simulink library "NeuroMuscularLibrary"  (R2019b)
settings: Solver=ode45  StartTime=0.0  StopTime=10.0  RelTol=1e-3  EnableMultiTasking=on
values from neighbouring files (symbols this model uses):
  a_18_19 = 116    [Prosthesis3R60Params.m]
  a_18_21 = 34    [Prosthesis3R60Params.m]
  a_2_3 = 18    [Prosthesis3R60Params.m]
  angle_offset = 0    [Prosthesis3R60Params.m]
  ankle_height = 0.08    [BodyMechParams.m]
  c = 0.05    [BodyMechParams.m]
  c_jointstop = 0.3 / (pi/180)    (= 17.1887338539)    [BodyMechParams.m]
  c_stance_comp_a0 = 885.0653    [Prosthesis3R60Params.m]
  c_stance_comp_a1 = 2.1443    [Prosthesis3R60Params.m]
  cg14 = 1/2*L14    (= 0.0475)    [Prosthesis3R60Params.m]
  cg25 = (5.45/11.05)*L25    (= 0.0379527149321)    [Prosthesis3R60Params.m]
  cg3 = (3.6/10.4)*L3    (= 0.0306346153846)    [Prosthesis3R60Params.m]
  d_fBall = 0.1    [BodyMechParams.m]
  d_fHeel = 0.05    [BodyMechParams.m]
  deltaLegAngleThr = 8*pi/180    (= 0.13962634016)    [CMGParams.m]
  DeltaThRef = 2e-3    (= 0.002)    [BodyMechParams.m]
  dt_visual = 0.001    [Prosthesis3R60Params.m]
  eref = 0.04    [BodyMechParams.m]
  Fmax = 4000    [MuscleEnergyTest.m]
  FmaxGLU = 1500    [BodyMechParams.m]
  footBallToAnkleDist = 0.16    [BodyMechParams.m]
  footBallToCenterDist = footLength/2    (= 0.1)    [BodyMechParams.m]
  footBallToHeelDist = footLength    (= 0.2)    [BodyMechParams.m]
  footCenterToCGDist = 0.14 - footBallToCenterDist    (= 0.04)    [BodyMechParams.m]
  footInertia = 0.005    [BodyMechParams.m]
  footLength = 0.2    [BodyMechParams.m]
  footMass = 1.25    [BodyMechParams.m]
  FT = 20    [MuscleEnergyTest.m]
  FT_GLU = 47.6    [BodyMechParams.m]
  g = 9.80665    [BodyMechParams.m]
  groundTheta = [atan(diff(groundZ)./diff(groundX)), 0]    [generateGround.m]
  groundZ = groundZ * stepSize/(largestStep+eps)    [generateGround.m]
  hatCenterToCGDist = 0.35 - hatHipToCenterDistLen    (= -0.05)    [BodyMechParams.m]
  hatHipToCenterDistLen = hatLength/2    (= 0.4)    [BodyMechParams.m]
  hatInertia = 3    [BodyMechParams.m]
  hatLeftHipToCenterDistWidth = .15    (= 0.15)    [BodyMechParams.m]
  hatLength = 0.8    [BodyMechParams.m]
  hatMass = 53.5    [BodyMechParams.m]
  hatThickness = 0.2    [BodyMechParams.m]
  hatWidth = 0.4    [BodyMechParams.m]
  J1011 = (4130)*1e-9    (= 4.13e-06)    [Prosthesis3R60Params.m]
  J1415 = (1.18*1e5)*1e-9    (= 0.000118)    [Prosthesis3R60Params.m]
  J18192021 = (6.86*1e4)*1e-9    (= 6.86e-05)    [Prosthesis3R60Params.m]
  J2526 = (3.59*1e4)*1e-9    (= 3.59e-05)    [Prosthesis3R60Params.m]
  J3467 = (25.96*1e4)*1e-9    (= 0.0002596)    [Prosthesis3R60Params.m]
  K = 5    [BodyMechParams.m]
  k_gn = k_gn/2    (= 39226.6)    [BodyMechParams.m]
  k_gt = k_gt/2    (= 39226.6)    [BodyMechParams.m]
  k_pressure = hatMass * g / DeltaThRef    (= 262327.8875)    [BodyMechParams.m]
  k_stance = 130000    [Prosthesis3R60Params.m]
  k_swing = 18750    [Prosthesis3R60Params.m]
  L0_stance = 0.08925    [Prosthesis3R60Params.m]
  L0_swing = 0.0896    [Prosthesis3R60Params.m]
  L10 = 7.9*1e-3    (= 0.0079)    [Prosthesis3R60Params.m]
  L11 = 3.3*1e-3    (= 0.0033)    [Prosthesis3R60Params.m]
  L14 = 95*1e-3    (= 0.095)    [Prosthesis3R60Params.m]
  L15 = 8.2*1e-3    (= 0.0082)    [Prosthesis3R60Params.m]
  L18 = 25.1*1e-3    (= 0.0251)    [Prosthesis3R60Params.m]
  L19 = 17.7*1e-3    (= 0.0177)    [Prosthesis3R60Params.m]
  L20 = 26*1e-3    (= 0.026)    [Prosthesis3R60Params.m]
  L21 = 1.7*1e-3    (= 0.0017)    [Prosthesis3R60Params.m]
  L25 = 76.95*1e-3    (= 0.07695)    [Prosthesis3R60Params.m]
  L26 = 2.8*1e-3    (= 0.0028)    [Prosthesis3R60Params.m]
  L3 = 88.5*1e-3    (= 0.0885)    [Prosthesis3R60Params.m]
  L4 = 1.7*1e-3    (= 0.0017)    [Prosthesis3R60Params.m]
  L6 = 40.25*1e-3    (= 0.04025)    [Prosthesis3R60Params.m]
  L7 = 14.9*1e-3    (= 0.0149)    [Prosthesis3R60Params.m]
  leg_l = [(thighLength - ankle_height/2) (shankLength - ankle_height/2)]    [BodyMechParams.m]
  legAngleSpeedMax = 10    [CMGParams.m]
  lopt = 0.055    [MuscleEnergyTest.m]
  loptBFSH = 0.12    [BodyMechParams.m]
  loptGAS = 0.05    [BodyMechParams.m]
  loptGLU = 0.11    [BodyMechParams.m]
  loptHAB = 0.09    [BodyMechParams.m]
  loptHAD = 0.10    (= 0.1)    [BodyMechParams.m]
  loptHAM = 0.10    (= 0.1)    [BodyMechParams.m]
  loptHFL = 0.11    [BodyMechParams.m]
  loptRF = 0.08    [BodyMechParams.m]
  loptSOL = 0.04    [BodyMechParams.m]
  loptTA = 0.06    [BodyMechParams.m]
  loptVAS = 0.08    [BodyMechParams.m]
  lslack = 0.245    [MuscleEnergyTest.m]
  lslackBFSH = 0.10    (= 0.1)    [BodyMechParams.m]
  lslackGAS = 0.40    (= 0.4)    [BodyMechParams.m]
  lslackGLU = 0.13    [BodyMechParams.m]
  lslackHAB = 0.07    [BodyMechParams.m]
  lslackHAD = 0.18    [BodyMechParams.m]
  lslackHAM = 0.31    [BodyMechParams.m]
  lslackHFL = 0.10    (= 0.1)    [BodyMechParams.m]
  lslackRF = 0.35    [BodyMechParams.m]
  lslackSOL = 0.26    [BodyMechParams.m]
  lslackTA = 0.24    [BodyMechParams.m]
  lslackVAS = 0.23    [BodyMechParams.m]
  m1011 = 49.5*1e-3    (= 0.0495)    [Prosthesis3R60Params.m]
  m1415 = 123.8*1e-3    (= 0.1238)    [Prosthesis3R60Params.m]
  m18192021 = 196.6*1e-3    (= 0.1966)    [Prosthesis3R60Params.m]
  m2526 = 58.3*1e-3    (= 0.0583)    [Prosthesis3R60Params.m]
  m3467 = 253.3*1e-3    (= 0.2533)    [Prosthesis3R60Params.m]
  mu_slide = 0.8    [BodyMechParams.m]
  mu_stick = 0.9    [BodyMechParams.m]
  N = 1.5    [BodyMechParams.m]    (also in cmaes.m = size(x,1); mergeCompareEnergyCosts.m = {S.name})
  phiKneeUpLimit = 5*pi/180    (= 0.0872664625997)    [BodyMechParams.m]
  phimaxGASa = (100-90)*pi/180    (= 0.174532925199)    [BodyMechParams.m]
  phimaxGASk = (180-140)*pi/180    (= 0.698131700798)    [BodyMechParams.m]
  phimaxRFk = (180-165)*pi/180    (= 0.261799387799)    [BodyMechParams.m]
  phimaxSOL = (100-90)*pi/180    (= 0.174532925199)    [BodyMechParams.m]
  phimaxTA = (80-90)*pi/180    (= -0.174532925199)    [BodyMechParams.m]
  phimaxVAS = (180-165)*pi/180    (= 0.261799387799)    [BodyMechParams.m]
  phirefBFSH = (180-160)*pi/180    (= 0.349065850399)    [BodyMechParams.m]
  phirefGASa = (80-90)*pi/180    (= -0.174532925199)    [BodyMechParams.m]
  phirefGASk = (180-165)*pi/180    (= 0.261799387799)    [BodyMechParams.m]
  phirefGLU = (120-180)*pi/180    (= -1.0471975512)    [BodyMechParams.m]
  phirefHAB = 10*pi/180    (= 0.174532925199)    [BodyMechParams.m]
  phirefHAD = 15*pi/180    (= 0.261799387799)    [BodyMechParams.m]
  phirefHAMh = (150-180)*pi/180    (= -0.523598775598)    [BodyMechParams.m]
  phirefHAMk = (180-180)*pi/180    (= 0)    [BodyMechParams.m]
  phirefHFL = (160-180)*pi/180    (= -0.349065850399)    [BodyMechParams.m]
  phirefRFh = (170-180)*pi/180    (= -0.174532925199)    [BodyMechParams.m]
  phirefRFk = (180-125)*pi/180    (= 0.959931088597)    [BodyMechParams.m]
  phirefSOL = (90-90)*pi/180    (= 0)    [BodyMechParams.m]
  ... (+64 more)
undefined symbols (not defined in the file or in its folder): ankleBackDriveGain, ankleCJointstop, ankleDgain, ankleFilterPID, ankleFilterSEA, ankleGearEff, ankleGearRatio, ankleIgain, ankleInitialAngle, ankleInputMass, ankleIntCoulomb, ankleIntDamping, ankleIntStatic, ankleParallelSpringDamping, ankleParallelSpringOffset, ankleParallelSpringStiffness, anklePgain, anklePlantarLimit, ankleSEADamping, ankleSEAStiffness, ankleTendonMass, ankleWMaxJointstop, D12_F, D12_S, D12_T, D12z_T, D13_F, D1G_F, D1G_HAT, D1G_S, D1G_T, D1Gy_F, DeltaS, DeltaSGLU, DeltaSHFL, dryFrictionDamping, dryFrictionStiffness, dryFrictionVelThresh, footMassp, FourBarL1, FourBarL3, GainDphiHATGLUst, GainDphiHATHABst, GainDphiHATHADst, GainDphiHATHFLst, GainFGASst, GainFGLUst, GainFHABst, GainFHAMst, GainFSOLst, GainFSOLTAst, GainFVASst, GainGAS, GainGLU, GainGLUswing, GainHAM, GainHAMHFL ... (+194)
libraries: sm_lib x332, nesl_utility x156, simulink x33, dspswit3 x30, $bdroot x19, simulink_extras x7
(part 2 of 15)

== system NeuroMuscularLibrary/Foots1 ==
  Brick Solid : sm_lib/Body Elements/Brick Solid  GraphicAmbientColor=[0.15 0.15 0.15 1.0]  BasedOnType=Density  BrickDimensions=[D13_F ankle_height d_fBall]  BrickDimensionUnits=m  CenterOfMass=[0 0 0]  CenterOfMassUnits=m  GraphicDiffuseColor=[0.5 0.5 0.5]  Density=0  DensityUnits=kg/m^3  DoExposeReferenceFrame=on  GraphicEmissiveColor=[0.0 0.0 0.0 1.0]  ExportEntireGeometry=off  SerializedFrames=<Frames/>  MarkerShape=Sphere  MarkerSize=10  GraphicType=FromGeometry  InertiaType=CalculateFromGeometry  Mass=1  MassUnits=kg  MomentsOfInertia=[1 1 1]  MomentsOfInertiaUnits=kg*m^2  GraphicOpacity=1.0  ProductsOfInertia=[0 0 0]  ProductsOfInertiaUnits=kg*m^2  GraphicShininess=75  GraphicSpecularColor=[0.5 0.5 0.5 1.0]  GraphicVisPropType=SimpleVisualProperties
  CS{1,5..6,9..10} (5 alike) : sm_lib/Frames and Transforms/Rigid Transform  TranslationMethod=None  TranslationStandardOffset=0  TranslationLengthUnit=m  TranslationStandardAxis=+Z  TranslationCartesianOffset=[0 0 0]  TranslationROffset=0  TranslationROffsetUnits=m  TranslationZOffset=0  TranslationZOffsetUnits=m  TranslationThetaOffset=0  TranslationThetaOffsetUnits=deg  RotationMethod=None  RotationAngleUnits=deg  RotationStandardAxis=+Z  RotationAngle=0.0  RotationArbitraryAxis=[0 0 1]  FollAlignAxisA=+X  BaseAlignAxisA=+Y  FollAlignAxisB=+Y  BaseAlignAxisB=+Z  RotationSequenceAxes=FollowerAxes  RotationSequence=XYX  RotationSequenceAngles=[0 0 0]  RotationSequenceAnglesUnits=deg  RotationMatrix=[1 0 0; 0 1 0; 0 0 1]
  CS2_to_ankle : sm_lib/Frames and Transforms/Rigid Transform  TranslationMethod=Cartesian  TranslationStandardOffset=0  TranslationLengthUnit=m  TranslationStandardAxis=+Z  TranslationCartesianOffset=[-D12_F ankle_height 0]  TranslationROffset=0  TranslationROffsetUnits=m  TranslationZOffset=0  TranslationZOffsetUnits=m  TranslationThetaOffset=0  TranslationThetaOffsetUnits=deg  RotationMethod=None  RotationAngleUnits=deg  RotationStandardAxis=+Z  RotationAngle=0.0  RotationArbitraryAxis=[0 0 1]  FollAlignAxisA=+X  BaseAlignAxisA=+Y  FollAlignAxisB=+Y  BaseAlignAxisB=+Z  RotationSequenceAxes=FollowerAxes  RotationSequence=XYX  RotationSequenceAngles=[0 0 0]  RotationSequenceAnglesUnits=deg  RotationMatrix=[1 0 0; 0 1 0; 0 0 1]
  CS3 : sm_lib/Frames and Transforms/Rigid Transform  TranslationMethod=Cartesian  TranslationStandardOffset=0  TranslationLengthUnit=m  TranslationStandardAxis=+Z  TranslationCartesianOffset=[0 0 -d_fBall/2]  TranslationROffset=0  TranslationROffsetUnits=m  TranslationZOffset=0  TranslationZOffsetUnits=m  TranslationThetaOffset=0  TranslationThetaOffsetUnits=deg  RotationMethod=None  RotationAngleUnits=deg  RotationStandardAxis=+Z  RotationAngle=0.0  RotationArbitraryAxis=[0 0 1]  FollAlignAxisA=+X  BaseAlignAxisA=+Y  FollAlignAxisB=+Y  BaseAlignAxisB=+Z  RotationSequenceAxes=FollowerAxes  RotationSequence=XYX  RotationSequenceAngles=[0 0 0]  RotationSequenceAnglesUnits=deg  RotationMatrix=[1 0 0; 0 1 0; 0 0 1]
  CS4 : sm_lib/Frames and Transforms/Rigid Transform  TranslationMethod=Cartesian  TranslationStandardOffset=0  TranslationLengthUnit=m  TranslationStandardAxis=+Z  TranslationCartesianOffset=[0 0 d_fBall/2]  TranslationROffset=0  TranslationROffsetUnits=m  TranslationZOffset=0  TranslationZOffsetUnits=m  TranslationThetaOffset=0  TranslationThetaOffsetUnits=deg  RotationMethod=None  RotationAngleUnits=deg  RotationStandardAxis=+Z  RotationAngle=0.0  RotationArbitraryAxis=[0 0 1]  FollAlignAxisA=+X  BaseAlignAxisA=+Y  FollAlignAxisB=+Y  BaseAlignAxisB=+Z  RotationSequenceAxes=FollowerAxes  RotationSequence=XYX  RotationSequenceAngles=[0 0 0]  RotationSequenceAnglesUnits=deg  RotationMatrix=[1 0 0; 0 1 0; 0 0 1]
  CS7 : sm_lib/Frames and Transforms/Rigid Transform  TranslationMethod=Cartesian  TranslationStandardOffset=0  TranslationLengthUnit=m  TranslationStandardAxis=+Z  TranslationCartesianOffset=[-D13_F 0 -d_fHeel/2]  TranslationROffset=0  TranslationROffsetUnits=m  TranslationZOffset=0  TranslationZOffsetUnits=m  TranslationThetaOffset=0  TranslationThetaOffsetUnits=deg  RotationMethod=None  RotationAngleUnits=deg  RotationStandardAxis=+Z  RotationAngle=0.0  RotationArbitraryAxis=[0 0 1]  FollAlignAxisA=+X  BaseAlignAxisA=+Y  FollAlignAxisB=+Y  BaseAlignAxisB=+Z  RotationSequenceAxes=FollowerAxes  RotationSequence=XYX  RotationSequenceAngles=[0 0 0]  RotationSequenceAnglesUnits=deg  RotationMatrix=[1 0 0; 0 1 0; 0 0 1]
  CS8 : sm_lib/Frames and Transforms/Rigid Transform  TranslationMethod=Cartesian  TranslationStandardOffset=0  TranslationLengthUnit=m  TranslationStandardAxis=+Z  TranslationCartesianOffset=[-D13_F 0 d_fHeel/2]  TranslationROffset=0  TranslationROffsetUnits=m  TranslationZOffset=0  TranslationZOffsetUnits=m  TranslationThetaOffset=0  TranslationThetaOffsetUnits=deg  RotationMethod=None  RotationAngleUnits=deg  RotationStandardAxis=+Z  RotationAngle=0.0  RotationArbitraryAxis=[0 0 1]  FollAlignAxisA=+X  BaseAlignAxisA=+Y  FollAlignAxisB=+Y  BaseAlignAxisB=+Z  RotationSequenceAxes=FollowerAxes  RotationSequence=XYX  RotationSequenceAngles=[0 0 0]  RotationSequenceAnglesUnits=deg  RotationMatrix=[1 0 0; 0 1 0; 0 0 1]
  Inertia : sm_lib/Body Elements/Inertia  InertiaType=Custom  Mass=m_F  MassUnits=kg  CenterOfMass=[0 0 0]  CenterOfMassUnits=m  MomentsOfInertia=[Inx_F Iny_F In_F]  MomentsOfInertiaUnits=kg*m^2  ProductsOfInertia=[0 0 0]  ProductsOfInertiaUnits=kg*m^2  GraphicType=None  MarkerShape=Inertia  MarkerSize=20  GraphicVisPropType=SimpleVisualProperties  GraphicDiffuseColor=[0.5 0.5 0.5]  GraphicSpecularColor=[0.5 0.5 0.5 1.0]  GraphicAmbientColor=[0.15 0.15 0.15 1.0]  GraphicEmissiveColor=[0.0 0.0 0.0 1.0]  GraphicShininess=75  GraphicOpacity=1.0
  Mux{,1..4} (5 alike) : Mux  Inputs=3
  PS-Simulink Converter{,1..14} (15 alike) : nesl_utility/PS-Simulink Converter  PhysicalDomain=network_engine_domain  SubClassName=ps_output  LeftPortType=input  RightPortType=output  PseudoPeriodic=off  Frequencies=[]  Unit=m  AffineConversion=off
  Reference Frame : sm_lib/Frames and Transforms/Reference Frame
  TO: X-forward Y-up Z-lateral : sm_lib/Frames and Transforms/Rigid Transform  TranslationMethod=StandardAxis  TranslationStandardOffset=D12z_T/2  TranslationLengthUnit=m  TranslationStandardAxis=+Y  TranslationCartesianOffset=[0 0 0]  TranslationROffset=0  TranslationROffsetUnits=m  TranslationZOffset=0  TranslationZOffsetUnits=m  TranslationThetaOffset=0  TranslationThetaOffsetUnits=deg  RotationMethod=AlignedAxes  RotationAngleUnits=deg  RotationStandardAxis=+Z  RotationAngle=0  RotationArbitraryAxis=[0 0 1]  FollAlignAxisA=+Z  BaseAlignAxisA=-Y  FollAlignAxisB=+X  BaseAlignAxisB=+X  RotationSequenceAxes=FollowerAxes  RotationSequence=XYX  RotationSequenceAngles=[0 0 0]  RotationSequenceAnglesUnits=deg  RotationMatrix=[1 0 0; 0 1 0; 0 0 1]
  To CG : sm_lib/Frames and Transforms/Rigid Transform  TranslationMethod=Cartesian  TranslationStandardOffset=0  TranslationLengthUnit=m  TranslationStandardAxis=+Z  TranslationCartesianOffset=[-D1G_F D1Gy_F 0]  TranslationROffset=0  TranslationROffsetUnits=m  TranslationZOffset=0  TranslationZOffsetUnits=m  TranslationThetaOffset=0  TranslationThetaOffsetUnits=deg  RotationMethod=None  RotationAngleUnits=deg  RotationStandardAxis=+Z  RotationAngle=0.0  RotationArbitraryAxis=[0 0 1]  FollAlignAxisA=+X  BaseAlignAxisA=+Y  FollAlignAxisB=+Y  BaseAlignAxisB=+Z  RotationSequenceAxes=FollowerAxes  RotationSequence=XYX  RotationSequenceAngles=[0 0 0]  RotationSequenceAnglesUnits=deg  RotationMatrix=[1 0 0; 0 1 0; 0 0 1]
  To center : sm_lib/Frames and Transforms/Rigid Transform  TranslationMethod=Cartesian  TranslationStandardOffset=0  TranslationLengthUnit=m  TranslationStandardAxis=+Z  TranslationCartesianOffset=[-D13_F/2 ankle_height/2 0]  TranslationROffset=0  TranslationROffsetUnits=m  TranslationZOffset=0  TranslationZOffsetUnits=m  TranslationThetaOffset=0  TranslationThetaOffsetUnits=deg  RotationMethod=None  RotationAngleUnits=deg  RotationStandardAxis=+Z  RotationAngle=0.0  RotationArbitraryAxis=[0 0 1]  FollAlignAxisA=+X  BaseAlignAxisA=+Y  FollAlignAxisB=+Y  BaseAlignAxisB=+Z  RotationSequenceAxes=FollowerAxes  RotationSequence=XYX  RotationSequenceAngles=[0 0 0]  RotationSequenceAnglesUnits=deg  RotationMatrix=[1 0 0; 0 1 0; 0 0 1]
  Transform Sensor{,1..4} (5 alike) : sm_lib/Frames and Transforms/Transform Sensor  MeasurementFrame=NonRotatingBase  SenseAngle=off  SenseAxis=off  SenseAngle1=off  SenseAngle2=off  SenseAngle3=off  SenseQ=off  SenseR=off  SenseOmegaX=off  SenseOmegaY=off  SenseOmegaZ=off  SenseOmega1=off  SenseOmega2=off  SenseOmega3=off  SenseQDot=off  SenseRDot=off  SenseAlphaX=off  SenseAlphaY=off  SenseAlphaZ=off  SenseAlpha1=off  SenseAlpha2=off  SenseAlpha3=off  SenseQDDot=off  SenseRDDot=off  SenseX=on  SenseY=on  SenseZ=on  SenseRad=off  SenseAzim=off  SenseDist=off  SenseInc=off  SenseXDot=off  SenseYDot=off  SenseZDot=off  SenseRadDot=off  SenseAzimDot=off  SenseDistDot=off  SenseIncDot=off  SenseXDDot=off  SenseYDDot=off  SenseZDDot=off  SenseRadDDot=off  SenseAzimDDot=off  SenseDistDDot=off  SenseIncDDot=off
  World Frame : sm_lib/Frames and Transforms/World Frame
  ankle : PMIOPort  Side=Right
  LLHeel Cnt : PMIOPort  Port=2  Side=Left
  LMHeel Cnt : PMIOPort  Port=3  Side=Left
  LMBall Cnt : PMIOPort  Port=4  Side=Left
  LLBall Cnt : PMIOPort  Port=5  Side=Left
  World : PMIOPort  Port=6  Side=Left
  LMBall Cnt pos : Outport
  LLBall Cnt pos : Outport  Port=2
  LMHeel Cnt pos : Outport  Port=3
  LLHeel Cnt pos : Outport  Port=4
  CG pos : Outport  Port=5
  wires:
  PS-Simulink Converter5/1 -> Mux1/3
  PS-Simulink Converter4/1 -> Mux1/2
  PS-Simulink Converter3/1 -> Mux1/1
  PS-Simulink Converter7/1 -> Mux2/2
  PS-Simulink Converter8/1 -> Mux2/1
  PS-Simulink Converter9/1 -> Mux3/3
  PS-Simulink Converter10/1 -> Mux3/2
  Mux3/1 -> LLHeel Cnt pos/1
  PS-Simulink Converter11/1 -> Mux3/1
  Mux2/1 -> LMHeel Cnt pos/1
  PS-Simulink Converter6/1 -> Mux2/3
  Mux1/1 -> LLBall Cnt pos/1
  Mux/1 -> LMBall Cnt pos/1
  PS-Simulink Converter1/1 -> Mux/3
  PS-Simulink Converter2/1 -> Mux/2
  PS-Simulink Converter/1 -> Mux/1
  PS-Simulink Converter12/1 -> Mux4/1
  PS-Simulink Converter13/1 -> Mux4/2
  PS-Simulink Converter14/1 -> Mux4/3
  Mux4/1 -> CG pos/1
  connections:
  TO: X-forward Y-up Z-lateral/LConn1 -- World Frame/RConn1
  Reference Frame/RConn1 -- Transform Sensor1/LConn1 -- Transform Sensor/LConn1 -- Transform Sensor2/LConn1 -- Transform Sensor4/LConn1 -- Transform Sensor3/LConn1 -- TO: X-forward Y-up Z-lateral/RConn1
  Brick Solid/RConn1 -- To center/RConn1
  PS-Simulink Converter5/LConn1 -- Transform Sensor1/RConn4
  PS-Simulink Converter4/LConn1 -- Transform Sensor1/RConn3
  PS-Simulink Converter3/LConn1 -- Transform Sensor1/RConn2
  CS7/LConn1 -- CS8/LConn1 -- CS4/LConn1 -- CS2_to_ankle/LConn1 -- CS3/LConn1 -- To center/LConn1 -- CS1/RConn1 -- To CG/LConn1
  Transform Sensor3/RConn3 -- PS-Simulink Converter10/LConn1
  Transform Sensor2/RConn3 -- PS-Simulink Converter7/LConn1
  Transform Sensor3/RConn2 -- PS-Simulink Converter11/LConn1
  Transform Sensor2/RConn4 -- PS-Simulink Converter6/LConn1
  Transform Sensor3/RConn4 -- PS-Simulink Converter9/LConn1
  Transform Sensor2/RConn2 -- PS-Simulink Converter8/LConn1
  Transform Sensor/RConn4 -- PS-Simulink Converter1/LConn1
  Transform Sensor/RConn3 -- PS-Simulink Converter2/LConn1
  PS-Simulink Converter/LConn1 -- Transform Sensor/RConn2
  World/RConn1 -- CS1/LConn1
  To CG/RConn1 -- Transform Sensor4/RConn1 -- Inertia/RConn1
  LMHeel Cnt/RConn1 -- CS10/RConn1
  LLBall Cnt/RConn1 -- CS5/RConn1
  ankle/RConn1 -- CS2_to_ankle/RConn1
  LLHeel Cnt/RConn1 -- CS9/RConn1
  LMBall Cnt/RConn1 -- CS6/RConn1
  CS7/RConn1 -- Transform Sensor2/RConn1 -- CS10/LConn1
  CS8/RConn1 -- Transform Sensor3/RConn1 -- CS9/LConn1
  CS3/RConn1 -- Transform Sensor/RConn1 -- CS6/LConn1
  CS4/RConn1 -- Transform Sensor1/RConn1 -- CS5/LConn1
  PS-Simulink Converter12/LConn1 -- Transform Sensor4/RConn2
  PS-Simulink Converter14/LConn1 -- Transform Sensor4/RConn4
  PS-Simulink Converter13/LConn1 -- Transform Sensor4/RConn3

== system NeuroMuscularLibrary/Force Plate ==
  "GRF_Ball [N N] " : Inport
  GRF_Heel [N N] : Inport  Port=2
  Enable : EnablePort  StatesWhenEnabling=reset
  Fcn : Fcn  Expr=u(1)/(u(2)+eps)
  Mux : Mux  Inputs=3
  Mux1 : Mux  Inputs=2
  Selector : Selector  InputPortWidth=2  IndexOptions=Index vector (dialog)  Indices=2  OutputSizes=1
  Selector1 : Selector  InputPortWidth=2  IndexOptions=Index vector (dialog)  Indices=2  OutputSizes=1
  Sum1 : Sum
  GRFs : Outport  OutputWhenDisabled=reset  InitialOutput=0
  COP : Outport  Port=2  OutputWhenDisabled=reset  InitialOutput=0
  wires:
  Selector/1 -> Mux1/2
  Selector1/1 -> Mux1/1
  "GRF_Ball [N N] "/1 -> Sum1/1, Mux/1, Selector1/1
  GRF_Heel [N N]/1 -> Sum1/2, Mux/3
  Sum1/1 -> Mux/2, Selector/1
  Mux/1 -> GRFs/1
  Mux1/1 -> Fcn/1
  Fcn/1 -> COP/1

== system NeuroMuscularLibrary/Full Prosthesis ==
  note: positive: extension
      | negative: flexion
  note: positive: dorsiflexion
      | negative: plantarflexion
  Desired Knee Torque : Inport
  Desired Ankle Torque : Inport  Port=2
  Ankle  Joint : Subsystem
  Ankle Input Joint : Subsystem
  Ankle Input Link : Subsystem
      mask Display: image('ankleInputLinkThumb.png')
  Ankle Motor : Subsystem
  Ankle Motor Rotor : Subsystem
      mask Display: image('motorRotorThumb.png')
  Ankle Parallel Spring : Subsystem
  Ankle SEA Control : Subsystem
  Ankle Tendon : Subsystem
      mask Display: image('ankleTendonThumb.png')
  Foot : Subsystem
      mask Display: image('footThumb.png')
  Gain{,1..7} (8 alike) : Gain  Gain=-1
  Harmonic Drive/ Series Elastic Actuator : Subsystem
  Harmonic Drive/ Series Elastic Actuator1 : Subsystem
  Knee Joint : Subsystem
  Knee Motor : Subsystem
  Knee Motor Rotor : Subsystem
      mask Display: image('motorRotorThumb.png')
  Knee SEA Control : Subsystem
  Knee Stator : Subsystem
      mask Display: image('kneeStatorThumb.png')
  Mux : Mux  Inputs=3
  Mux1 : Mux
  Scope : Scope  NumInputPorts=3
  Scope2 : Scope  NumInputPorts=3
  Shank : Subsystem
      mask Display: image('shankThumb.png')
  Thigh : PMIOPort  Side=Left
  Knee Follwoer : PMIOPort  Port=2  Side=Left
  Ankle : PMIOPort  Port=3  Side=Right
  Ball : PMIOPort  Port=4  Side=Right
  Heel : PMIOPort  Port=5  Side=Right
  Knee Angle : Outport
  Knee Speed : Outport  Port=2
  Ankle Angle : Outport  Port=3
  Ankle Speed : Outport  Port=4
  Knee Stop Torque : Outport  Port=5
  Ankle Stop Torque : Outport  Port=6
  wires:
  Ankle  Joint/4(Ankle Stop Torque) -> Gain6/1
  Gain6/1 -> Ankle Stop Torque/1
  Knee Joint/5(Knee Stop Torque) -> Gain5/1
  Gain5/1 -> Knee Stop Torque/1
  Ankle SEA Control/2(Desired Actuator Torque) -> Mux1/3  "Desired Actuaor Torque"
  Mux1/1 -> Scope2/1
  Gain2/1 -> Ankle SEA Control/4(Desired Ankle Torque), Mux1/1  "Desired Ankle Torque"
  Harmonic Drive/ Series Elastic Actuator1/2(Torque on Load) -> Ankle Input Joint/1(Torque on Ankle Input), Mux1/4, Ankle SEA Control/3(Measured Torque)  "Measured Torque"
  Ankle Motor/1(Motor Torque) -> Harmonic Drive/ Series Elastic Actuator1/3(Motor Torque), Scope2/2  "Motor Torque"
  Ankle SEA Control/1(Motor Voltage) -> Ankle Motor/1(Voltage), Scope2/3  "Voltage"
  Gain7/1 -> Ankle Speed/1
  Gain1/1 -> Ankle Angle/1
  Knee Joint/4(Actual Torque) -> Mux/1  "Actual Torque"
  Knee Motor/2(Motor Angle) -> Harmonic Drive/ Series Elastic Actuator/2(Motor Angle)
  Knee Motor/3(Motor Speed) -> Harmonic Drive/ Series Elastic Actuator/1(Motor Speed), Knee SEA Control/1(Motor Speed)
  Knee Motor/1(Motor Torque) -> Harmonic Drive/ Series Elastic Actuator/3(Motor Torque), Scope/2  "Motor Torque"
  Harmonic Drive/ Series Elastic Actuator/1(Torque on Motor) -> Knee Motor/2(Net Motor Torque)
  Knee Joint/1(Shank Angle) -> Gain3/1, Harmonic Drive/ Series Elastic Actuator/4(Load Angle)
  Knee Joint/2(Shank Speed) -> Gain4/1, Knee Motor/3(Load Speed), Harmonic Drive/ Series Elastic Actuator/5(Load Speed)
  Knee SEA Control/1(Motor Voltage) -> Scope/3, Knee Motor/1(Voltage)  "Voltage"
  Knee Joint/3(Shank Acceleration) -> Knee SEA Control/2(Load Acceleration)
  Ankle Motor/2(Motor Angle) -> Harmonic Drive/ Series Elastic Actuator1/2(Motor Angle)
  Ankle Motor/3(Motor Speed) -> Ankle SEA Control/1(Motor Speed), Harmonic Drive/ Series Elastic Actuator1/1(Motor Speed)
  Ankle Input Joint/1(Ankle Input Angle) -> Ankle SEA Control/6(Ankle Input Angle), Harmonic Drive/ Series Elastic Actuator1/4(Load Angle)
  Harmonic Drive/ Series Elastic Actuator1/1(Torque on Motor) -> Ankle Motor/2(Net Motor Torque)
  Ankle Input Joint/3(Ankle Input Accel) -> Ankle SEA Control/2(Load Acceleration)
  Ankle Tendon/1(Angle) -> Ankle SEA Control/7(Tendon Angle)
  Ankle Input Joint/2(Ankle Input Speed) -> Ankle Motor/3(Load Speed), Harmonic Drive/ Series Elastic Actuator1/5(Load Speed)
  Mux/1 -> Scope/1
  Gain/1 -> Mux/3, Knee SEA Control/4(Desired Torque)  "Desired Torque"
  Harmonic Drive/ Series Elastic Actuator/2(" Torque on Load") -> Knee SEA Control/3(Measured Torque), Mux/2, Knee Joint/1(External Torque)  "Measured Torque"
  Ankle Parallel Spring/1(Parallel Spring Torque) -> Ankle  Joint/1(Torque on Ankle), Ankle SEA Control/5(Parallel Spring Torque)
  Desired Knee Torque/1 -> Gain/1
  Desired Ankle Torque/1 -> Gain2/1
  Gain3/1 -> Knee Angle/1
  Gain4/1 -> Knee Speed/1
  Ankle  Joint/1(Ankle Angle) -> Ankle Parallel Spring/1(Ankle Angle), Gain1/1, Ankle SEA Control/8(Ankle Angle)
  Ankle  Joint/2(Ankle Speed) -> Ankle Parallel Spring/2(Ankle Speed), Gain7/1
  Ankle  Joint/3(Actual Torque) -> Mux1/2
  connections:
  Thigh/RConn1 -- Knee Stator/RConn1
  Knee Stator/LConn1 -- Knee Motor/RConn1 -- Knee Joint/RConn1
  Knee Motor Rotor/RConn1 -- Knee Motor/LConn1
  Shank/RConn1 -- Knee Joint/LConn1 -- Knee Follwoer/RConn1
  Shank/LConn1 -- Ankle Motor/RConn1 -- Ankle Input Joint/RConn1
  Ankle Motor Rotor/RConn1 -- Ankle Motor/LConn1
  Ankle Input Link/RConn1 -- Ankle Input Joint/LConn1
  Ankle  Joint/LConn1 -- Shank/LConn2
  Foot/RConn1 -- Ankle/RConn1 -- Ankle  Joint/RConn1
  Ankle Tendon/LConn1 -- Ankle Input Link/LConn1
  Foot/LConn1 -- Ankle Tendon/RConn1
  Ball/RConn1 -- Foot/LConn2
  Heel/RConn1 -- Foot/RConn2

== system NeuroMuscularLibrary/GAS Link ==
  note: GAS Attachment
  Knee angle [rad] : Inport
  Ankle angle [rad] : Inport  Port=2
  Constant1 : Constant  Value=phimaxGASk
  Constant2 : Constant  Value=phirefGASk
  Constant3 : Constant  Value=phimaxGASa
  Constant4 : Constant  Value=lslackGAS+loptGAS
  Constant5 : Constant  Value=phirefGASa
  Demux : Demux  Outputs=2
  Demux1 : Demux  Outputs=2
  Gain1 : Gain  Gain=rGASkmax
  Gain2 : Gain  Gain=rGASamax
  Gain3 : Gain  Gain=phiScaleGASa
  Gain5 : Gain  Gain=phiScaleGASk
  Gain6 : Gain  Gain=phiScaleGASk
  Gain7 : Gain  Gain=rhoGASk/phiScaleGASk
  Gain8 : Gain  Gain=phiScaleGASa
  Gain9 : Gain  Gain=rhoGASa/phiScaleGASa
  Multiply : Gain  Gain=-1
  Mux : Mux  Inputs=2
  Mux1 : Mux  Inputs=2
  Sum1 : Sum  Inputs=-+
  Sum2 : Sum  Inputs=|+-
  Sum3 : Sum  Inputs=-+|
  Sum4 : Sum  Inputs=-+
  Sum5 : Sum  Inputs=-+-
  Sum6 : Sum  Inputs=|+-
  Sum7 : Sum  Inputs=-+|
  length change term : Trigonometry
  length change term1 : Trigonometry
  offset correction term : Trigonometry
  offset correction term1 : Trigonometry
  variable lever term : Trigonometry  Operator=cos
  variable lever term1 : Trigonometry  Operator=cos
  lmtu [m] : Outport
  leverKnee [m] : Outport  Port=2
  leverAnkle [m] : Outport  Port=3
  wires:
  Sum4/1 -> Mux1/1
  Gain8/1 -> offset correction term1/1
  Gain7/1 -> Sum5/1
  Demux1/2 -> leverAnkle [m]/1
  Constant4/1 -> Sum5/2
  Sum5/1 -> lmtu [m]/1
  Demux1/1 -> Gain9/1
  Demux/1 -> Multiply/1
  Mux1/1 -> Gain2/1
  Sum2/1 -> Gain6/1
  Gain2/1 -> Demux1/1
  offset correction term1/1 -> Sum4/1
  Gain6/1 -> offset correction term/1
  length change term1/1 -> Sum4/2
  variable lever term/1 -> Mux/2
  Constant5/1 -> Sum6/1
  Demux/2 -> leverKnee [m]/1
  Sum6/1 -> Gain8/1
  Gain1/1 -> Demux/1
  Mux/1 -> Gain1/1
  Sum1/1 -> Mux/1
  Constant3/1 -> Sum7/1, Sum6/2
  Sum7/1 -> Gain3/1
  Gain5/1 -> variable lever term/1, length change term/1
  offset correction term/1 -> Sum1/1
  variable lever term1/1 -> Mux1/2
  Constant1/1 -> Sum3/1, Sum2/2
  Gain9/1 -> Sum5/3
  Constant2/1 -> Sum2/1
  length change term/1 -> Sum1/2
  Gain3/1 -> variable lever term1/1, length change term1/1
  Sum3/1 -> Gain5/1
  Knee angle [rad]/1 -> Sum3/2
  Ankle angle [rad]/1 -> Sum7/2
  Multiply/1 -> Gain7/1

== system NeuroMuscularLibrary/GLU Link ==
  note: GLUTEUS Attachment
  hip angle [rad] : Inport
  Constant : Constant  Value=lslackGLU+loptGLU
  Constant1 : Constant  Value=rGLU
  Constant2 : Constant  Value=phirefGLU
  Gain2 : Gain  Gain=rhoGLU
  Product : Product  RndMeth=Zero
  Sum2 : Sum  Inputs=|+-
  Sum5 : Sum  Inputs=|+-
  lmtu [m] : Outport
  lever [m] : Outport  Port=2
  wires:
  Constant/1 -> Sum5/1
  Sum5/1 -> lmtu [m]/1
  Product/1 -> Gain2/1
  Constant2/1 -> Sum2/2
  Sum2/1 -> Product/1
  Constant1/1 -> Product/2, lever [m]/1
  Gain2/1 -> Sum5/2
  hip angle [rad]/1 -> Sum2/1

== system NeuroMuscularLibrary/Ground Contact Model ==
  note: 2D Ground Interaction Model
  Env : Inport
  " contact sensor" : simulink/Logic and Bit Operations/Compare To Zero  relop=<=  OutDataTypeStr=boolean
  2D Contact : Subsystem
  Demux : Demux  Outputs=2
  Demux2 : Demux  Outputs=[1 2 2]
  External Force and Torque : sm_lib/Forces and Torques/External Force and Torque  ForceResolutionFrame=World  EnableForceX=on  EnableForceY=off  EnableForceZ=on  EnableForce=off  TorqueResolutionFrame=AttachedFrame  EnableTorqueX=off  EnableTorqueY=off  EnableTorqueZ=off  EnableTorque=off
  Mux1 : Mux  Inputs=2
  Mux2 : Mux  Inputs=2
  PS-Simulink Converter : nesl_utility/PS-Simulink Converter  PhysicalDomain=network_engine_domain  SubClassName=ps_output  LeftPortType=input  RightPortType=output  PseudoPeriodic=off  Frequencies=[]  Unit=m  AffineConversion=off
  PS-Simulink Converter1 : nesl_utility/PS-Simulink Converter  PhysicalDomain=network_engine_domain  SubClassName=ps_output  LeftPortType=input  RightPortType=output  PseudoPeriodic=off  Frequencies=[]  Unit=m/s  AffineConversion=off
  PS-Simulink Converter2 : nesl_utility/PS-Simulink Converter  PhysicalDomain=network_engine_domain  SubClassName=ps_output  LeftPortType=input  RightPortType=output  PseudoPeriodic=off  Frequencies=[]  Unit=m  AffineConversion=off
  PS-Simulink Converter3 : nesl_utility/PS-Simulink Converter  PhysicalDomain=network_engine_domain  SubClassName=ps_output  LeftPortType=input  RightPortType=output  PseudoPeriodic=off  Frequencies=[]  Unit=m/s  AffineConversion=off
  Simulink-PS Converter : nesl_utility/Simulink-PS Converter  PhysicalDomain=network_engine_domain  SubClassName=ps_input  LeftPortType=input  RightPortType=output  PseudoPeriodic=off  Frequencies=[]  NoiseDistribution=none  NoiseParameters=[]  Unit=1  AffineConversion=off  FilteringAndDerivatives=zero  SimscapeFilterOrder=1  InputFilterTimeConstant=0.001  UdotUserProvided=1
  Simulink-PS Converter1 : nesl_utility/Simulink-PS Converter  PhysicalDomain=network_engine_domain  SubClassName=ps_input  LeftPortType=input  RightPortType=output  PseudoPeriodic=off  Frequencies=[]  NoiseDistribution=none  NoiseParameters=[]  Unit=1  AffineConversion=off  FilteringAndDerivatives=zero  SimscapeFilterOrder=1  InputFilterTimeConstant=0.001  UdotUserProvided=1
  Sum : Sum  Inputs=-+|
  Sum1 : Sum
  Transform Sensor : sm_lib/Frames and Transforms/Transform Sensor  MeasurementFrame=World  SenseAngle=off  SenseAxis=off  SenseAngle1=off  SenseAngle2=off  SenseAngle3=off  SenseQ=off  SenseR=off  SenseOmegaX=off  SenseOmegaY=off  SenseOmegaZ=off  SenseOmega1=off  SenseOmega2=off  SenseOmega3=off  SenseQDot=off  SenseRDot=off  SenseAlphaX=off  SenseAlphaY=off  SenseAlphaZ=off  SenseAlpha1=off  SenseAlpha2=off  SenseAlpha3=off  SenseQDDot=off  SenseRDDot=off  SenseX=on  SenseY=off  SenseZ=on  SenseRad=off  SenseAzim=off  SenseDist=off  SenseInc=off  SenseXDot=on  SenseYDot=off  SenseZDot=on  SenseRadDot=off  SenseAzimDot=off  SenseDistDot=off  SenseIncDot=off  SenseXDDot=off  SenseYDDot=off  SenseZDDot=off  SenseRadDDot=off  SenseAzimDDot=off  SenseDistDDot=off  SenseIncDDot=off
  World Frame : sm_lib/Frames and Transforms/World Frame
  Foot : PMIOPort  Side=Left
  Contact? : Outport
  GRF [N N] : Outport  Port=2
  wires:
  Demux/2 -> Simulink-PS Converter1/1
  Demux/1 -> Simulink-PS Converter/1
  Demux2/3 -> 2D Contact/2(nVec [m m])  "Normal Vector"
  Demux2/2 -> 2D Contact/1(RefPt [m m])  "Reference Point"
  Demux2/1 -> Sum/1  "Ground Height"
  Env/1 -> Demux2/1
  Mux2/1 -> 2D Contact/4(vVec [m/s m/s])
  2D Contact/2(FtVec [N N]) -> Sum1/2
  2D Contact/1(FnVec [N N]) -> Sum1/1
  Mux1/1 -> 2D Contact/3(pVec [m m])
  " contact sensor"/1 -> 2D Contact/Enable, Contact?/1
  PS-Simulink Converter1/1 -> Mux2/1
  PS-Simulink Converter/1 -> Mux1/1
  PS-Simulink Converter3/1 -> Mux2/2
  PS-Simulink Converter2/1 -> Sum/2, Mux1/2
  Sum/1 -> " contact sensor"/1
  Sum1/1 -> GRF [N N]/1, Demux/1
  connections:
  External Force and Torque/LConn1 -- Simulink-PS Converter/RConn1
  External Force and Torque/LConn2 -- Simulink-PS Converter1/RConn1
  Foot/RConn1 -- External Force and Torque/RConn1 -- Transform Sensor/RConn1
  Transform Sensor/LConn1 -- World Frame/RConn1
  Transform Sensor/RConn5 -- PS-Simulink Converter3/LConn1
  Transform Sensor/RConn4 -- PS-Simulink Converter1/LConn1
  Transform Sensor/RConn3 -- PS-Simulink Converter2/LConn1
  Transform Sensor/RConn2 -- PS-Simulink Converter/LConn1

== system NeuroMuscularLibrary/Ground Height Lookup ==
  LHeel : Inport
  LBall : Inport  Port=2
  RHeel : Inport  Port=3
  RBall : Inport  Port=4
  HATCG : Inport  Port=5
  Env Lookup : Subsystem
  Env Lookup1 : Subsystem
  Env Lookup2 : Subsystem
  Env Lookup3 : Subsystem
  Env Lookup4 : Subsystem
  Selector : Selector  InputPortWidth=5  IndexOptions=Index vector (dialog)  Indices=[1]  OutputSizes=1
  Selector{1..5} (5 alike) : Selector  InputPortWidth=3  IndexOptions=Index vector (dialog)  Indices=[1]  OutputSizes=1
  LHeelEnv : Outport  OutputWhenDisabled=reset  InitialOutput=0
  LBallEnv : Outport  Port=2  OutputWhenDisabled=reset  InitialOutput=0
  RHeelEnv : Outport  Port=3  OutputWhenDisabled=reset  InitialOutput=0
  RBallEnv : Outport  Port=4  OutputWhenDisabled=reset  InitialOutput=0
  HATGroundy : Outport  Port=5  OutputWhenDisabled=reset  InitialOutput=0
  wires:
  LHeel/1 -> Selector5/1
  LBall/1 -> Selector1/1
  RHeel/1 -> Selector3/1
  RBall/1 -> Selector4/1
  Selector5/1 -> Env Lookup/1(x)
  Env Lookup/1(Env) -> LHeelEnv/1
  Selector1/1 -> Env Lookup1/1(x)
  Env Lookup1/1(Env) -> LBallEnv/1
  Selector3/1 -> Env Lookup2/1(x)
  Selector4/1 -> Env Lookup3/1(x)
  Env Lookup2/1(Env) -> RHeelEnv/1
  Env Lookup3/1(Env) -> RBallEnv/1
  HATCG/1 -> Selector2/1
  Selector2/1 -> Env Lookup4/1(x)
  Env Lookup4/1(Env) -> Selector/1
  Selector/1 -> HATGroundy/1

== system NeuroMuscularLibrary/HAB Link ==
  note: HAB Attachment
  Hip roll angle [rad] : Inport
  Constant : Constant  Value=lslackHAB+loptHAB
  Constant1 : Constant  Value=rHAB
  Constant2 : Constant  Value=phirefHAB
  Gain2 : Gain  Gain=rhoHAB
  Product : Product  RndMeth=Zero
  Sum2 : Sum  Inputs=|+-
  Sum5 : Sum  Inputs=|+-
  lmtu [m] : Outport
  lever [m] : Outport  Port=2
  wires:
  Gain2/1 -> Sum5/2
  Constant1/1 -> lever [m]/1, Product/2
  Sum2/1 -> Product/1
  Constant2/1 -> Sum2/2
  Hip roll angle [rad]/1 -> Sum2/1
  Product/1 -> Gain2/1
  Sum5/1 -> lmtu [m]/1
  Constant/1 -> Sum5/1

== system NeuroMuscularLibrary/HAD Link ==
  note: HAD Attachment
  hip roll angle [rad] : Inport
  Constant : Constant  Value=lslackHAD+loptHAD
  Constant1 : Constant  Value=rHAD
  Constant2 : Constant  Value=phirefHAD
  Gain2 : Gain  Gain=rhoHAD
  Product : Product  RndMeth=Zero
  Sum2 : Sum  Inputs=|+-
  Sum5 : Sum  Inputs=|++
  lmtu [m] : Outport
  lever [m] : Outport  Port=2
  wires:
  Constant/1 -> Sum5/1
  Sum5/1 -> lmtu [m]/1
  Product/1 -> Gain2/1
  hip roll angle [rad]/1 -> Sum2/1
  Constant2/1 -> Sum2/2
  Sum2/1 -> Product/1
  Constant1/1 -> Product/2, lever [m]/1
  Gain2/1 -> Sum5/2

== system NeuroMuscularLibrary/HAM Link ==
  note: HAM Attachment
  hip angle : Inport
  knee angle : Inport  Port=2
  Constant1 : Constant  Value=rHAMk
  Constant10 : Constant  Value=phirefHAMh
  Constant2 : Constant  Value=phirefHAMk
  Constant3 : Constant  Commented=on  Value=rHAMh
  Constant4 : Constant  Commented=on  Value=lslackHAM+loptHAM
  Constant5 : Constant  Commented=on  Value=phirefHAMh
  Constant6 : Constant  Commented=on  Value=phirefHAMk
  Constant7 : Constant  Commented=on  Value=phimaxHAMk  VectorParams1D=off
  Constant8 : Constant  Value=rHAMh
  Constant9 : Constant  Value=lslackHAM+loptHAM
  Demux1 : Demux  Commented=on  Outputs=2
  Gain1 : Gain  Gain=rhoHAMh
  Gain2 : Gain  Commented=on  Gain=rhoHAMh
  Gain3 : Gain  Commented=on  Gain=rHAMk
  Gain4 : Gain  Commented=on  Gain=rhoHAMk
  Gain5 : Gain  Gain=rhoHAMk
  Multiply : Gain  Gain=-1
  Mux1 : Mux  Commented=on  Inputs=2
  Product : Product  Commented=on  RndMeth=Zero
  Product1 : Product  RndMeth=Zero
  Product2 : Product  RndMeth=Zero
  Sum1 : Sum  Inputs=|+-
  Sum2 : Sum  Inputs=|+-
  Sum3 : Sum  Inputs=-+-
  Sum4 : Sum  Commented=on  Inputs=|+-
  Sum5 : Sum  Commented=on  Inputs=-++
  Sum7 : Sum  Commented=on  Inputs=|+-
  Sum8 : Sum  Commented=on  Inputs=-+|
  Sum9 : Sum  Commented=on  Inputs=+-
  length change term ankle : Trigonometry  Commented=on
  offset correction term ankle : Trigonometry  Commented=on
  variable lever term ankle : Trigonometry  Commented=on  Operator=cos
  lmtu [m] : Outport
  hip lever [m] : Outport  Port=2
  knee lever [m] : Outport  Port=3
  wires:
  Constant5/1 -> Sum4/2
  Sum4/1 -> Product/1
  Constant3/1 -> Product/2
  Product/1 -> Gain2/1
  Sum5/1 -> ?
  variable lever term ankle/1 -> Mux1/2
  Demux1/2 -> ?
  Sum8/1 -> variable lever term ankle/1, length change term ankle/1
  Constant7/1 -> Sum8/1, Sum7/2
  Sum7/1 -> offset correction term ankle/1
  Constant6/1 -> Sum7/1
  length change term ankle/1 -> Sum9/2
  offset correction term ankle/1 -> Sum9/1
  Sum9/1 -> Mux1/1
  Constant4/1 -> Sum5/2
  Mux1/1 -> Gain3/1
  Gain3/1 -> Demux1/1
  Demux1/1 -> Gain4/1
  Gain4/1 -> Sum5/3
  Gain2/1 -> Sum5/1
  ? -> Sum4/1
  ? -> Sum8/2
  Product2/1 -> Multiply/1
  Sum1/1 -> Product2/1
  Constant1/1 -> knee lever [m]/1, Product2/2
  Product1/1 -> Gain1/1
  Constant2/1 -> Sum1/2
  Sum3/1 -> lmtu [m]/1
  Gain1/1 -> Sum3/1
  Constant10/1 -> Sum2/2
  Constant8/1 -> hip lever [m]/1, Product1/2
  Constant9/1 -> Sum3/2
  Gain5/1 -> Sum3/3
  Sum2/1 -> Product1/1
  hip angle/1 -> Sum2/1
  knee angle/1 -> Sum1/1
  Multiply/1 -> Gain5/1

== system NeuroMuscularLibrary/HAT ==
  HAT CG : sm_lib/Frames and Transforms/Reference Frame
  HAT Center to CG : sm_lib/Frames and Transforms/Rigid Transform  TranslationMethod=Cartesian  TranslationStandardOffset=0  TranslationLengthUnit=m  TranslationStandardAxis=+Z  TranslationCartesianOffset=[0, hatCenterToCGDist, 0]  TranslationROffset=0  TranslationROffsetUnits=m  TranslationZOffset=0  TranslationZOffsetUnits=m  TranslationThetaOffset=0  TranslationThetaOffsetUnits=deg  RotationMethod=None  RotationAngleUnits=deg  RotationStandardAxis=+Z  RotationAngle=0  RotationArbitraryAxis=[0 0 1]  FollAlignAxisA=+X  BaseAlignAxisA=+Y  FollAlignAxisB=+Y  BaseAlignAxisB=+Z  RotationSequenceAxes=FollowerAxes  RotationSequence=XYX  RotationSequenceAngles=[0 0 0]  RotationSequenceAnglesUnits=deg  RotationMatrix=[1 0 0; 0 1 0; 0 0 1]
  HAT Center to Top : sm_lib/Frames and Transforms/Rigid Transform  TranslationMethod=StandardAxis  TranslationStandardOffset=hatLength/2  TranslationLengthUnit=m  TranslationStandardAxis=+Y  TranslationCartesianOffset=[0, 0, 0]  TranslationROffset=0  TranslationROffsetUnits=m  TranslationZOffset=0  TranslationZOffsetUnits=m  TranslationThetaOffset=0  TranslationThetaOffsetUnits=deg  RotationMethod=None  RotationAngleUnits=deg  RotationStandardAxis=+Z  RotationAngle=0  RotationArbitraryAxis=[0 0 1]  FollAlignAxisA=+X  BaseAlignAxisA=+Y  FollAlignAxisB=+Y  BaseAlignAxisB=+Z  RotationSequenceAxes=FollowerAxes  RotationSequence=XYX  RotationSequenceAngles=[0 0 0]  RotationSequenceAnglesUnits=deg  RotationMatrix=[1 0 0; 0 1 0; 0 0 1]
  Hip Solid : sm_lib/Body Elements/Brick Solid  GraphicAmbientColor=[0.15 0.15 0.15 1.0]  BasedOnType=Density  BrickDimensions=[hatThickness, hatLength, hatWidth]  BrickDimensionUnits=m  CenterOfMass=[0, 0, 0]  CenterOfMassUnits=m  GraphicDiffuseColor=[0.5 0.5 0.5]  Density=1000  DensityUnits=kg/(m^3)  DoExposeReferenceFrame=on  GraphicEmissiveColor=[0.0 0.0 0.0 1.0]  ExportEntireGeometry=off  SerializedFrames=<Frames/>  MarkerShape=Sphere  MarkerSize=10  GraphicType=FromGeometry  InertiaType=Custom  Mass=hatMass  MassUnits=kg  MomentsOfInertia=[0 0 0]  MomentsOfInertiaUnits=kg*m^2  GraphicOpacity=1.0  ProductsOfInertia=[0 0 0]  ProductsOfInertiaUnits=kg*m^2  GraphicShininess=75  GraphicSpecularColor=[0.5 0.5 0.5 1.0]  GraphicVisPropType=SimpleVisualProperties
  Inertia : sm_lib/Body Elements/Inertia  InertiaType=Custom  Mass=hatMass  MassUnits=kg  CenterOfMass=[0 0 0]  CenterOfMassUnits=m  MomentsOfInertia=[0 0 hatInertia]  MomentsOfInertiaUnits=kg*m^2  ProductsOfInertia=[0 0 0]  ProductsOfInertiaUnits=kg*m^2  GraphicType=None  MarkerShape=Inertia  MarkerSize=20  GraphicVisPropType=SimpleVisualProperties  GraphicDiffuseColor=[0.5 0.5 0.5]  GraphicSpecularColor=[0.5 0.5 0.5 1.0]  GraphicAmbientColor=[0.15 0.15 0.15 1.0]  GraphicEmissiveColor=[0.0 0.0 0.0 1.0]  GraphicShininess=75  GraphicOpacity=1.0
  Left Hip to Center : sm_lib/Frames and Transforms/Rigid Transform  TranslationMethod=Cartesian  TranslationStandardOffset=0  TranslationLengthUnit=m  TranslationStandardAxis=+Z  TranslationCartesianOffset=[0, hatHipToCenterDistLen, hatLeftHipToCenterDistWidth]  TranslationROffset=0  TranslationROffsetUnits=m  TranslationZOffset=0  TranslationZOffsetUnits=m  TranslationThetaOffset=0  TranslationThetaOffsetUnits=deg  RotationMethod=None  RotationAngleUnits=deg  RotationStandardAxis=+Z  RotationAngle=0  RotationArbitraryAxis=[0 0 1]  FollAlignAxisA=+X  BaseAlignAxisA=+Y  FollAlignAxisB=+Y  BaseAlignAxisB=+Z  RotationSequenceAxes=FollowerAxes  RotationSequence=XYX  RotationSequenceAngles=[0 0 0]  RotationSequenceAnglesUnits=deg  RotationMatrix=[1 0 0; 0 1 0; 0 0 1]
  Left Hip to Right Hip : sm_lib/Frames and Transforms/Rigid Transform  TranslationMethod=Cartesian  TranslationStandardOffset=0  TranslationLengthUnit=m  TranslationStandardAxis=+Z  TranslationCartesianOffset=[0 0 2*hatLeftHipToCenterDistWidth]  TranslationROffset=0  TranslationROffsetUnits=m  TranslationZOffset=0  TranslationZOffsetUnits=m  TranslationThetaOffset=0  TranslationThetaOffsetUnits=deg  RotationMethod=None  RotationAngleUnits=deg  RotationStandardAxis=+Z  RotationAngle=0  RotationArbitraryAxis=[0 0 1]  FollAlignAxisA=+X  BaseAlignAxisA=+Y  FollAlignAxisB=+Y  BaseAlignAxisB=+Z  RotationSequenceAxes=FollowerAxes  RotationSequence=XYX  RotationSequenceAngles=[0 0 0]  RotationSequenceAnglesUnits=deg  RotationMatrix=[1 0 0; 0 1 0; 0 0 1]
  Mux : Mux  Inputs=2
  PS-Simulink Converter : nesl_utility/PS-Simulink Converter  PhysicalDomain=network_engine_domain  SubClassName=ps_output  LeftPortType=input  RightPortType=output  PseudoPeriodic=off  Frequencies=[]  Unit=1  AffineConversion=off
  PS-Simulink Converter1 : nesl_utility/PS-Simulink Converter  PhysicalDomain=network_engine_domain  SubClassName=ps_output  LeftPortType=input  RightPortType=output  PseudoPeriodic=off  Frequencies=[]  Unit=1  AffineConversion=off
  To: X-forward Y-Lateral Z-up : sm_lib/Frames and Transforms/Rigid Transform  TranslationMethod=None  TranslationStandardOffset=0  TranslationLengthUnit=m  TranslationStandardAxis=+Z  TranslationCartesianOffset=[0, hatHipToCenterDistLen, -hatLeftHipToCenterDistWidth]  TranslationROffset=0  TranslationROffsetUnits=m  TranslationZOffset=0  TranslationZOffsetUnits=m  TranslationThetaOffset=0  TranslationThetaOffsetUnits=deg  RotationMethod=AlignedAxes  RotationAngleUnits=deg  RotationStandardAxis=+Z  RotationAngle=0  RotationArbitraryAxis=[0 0 1]  FollAlignAxisA=+X  BaseAlignAxisA=+X  FollAlignAxisB=+Z  BaseAlignAxisB=+Y  RotationSequenceAxes=FollowerAxes  RotationSequence=XYX  RotationSequenceAngles=[0 0 0]  RotationSequenceAnglesUnits=deg  RotationMatrix=[1 0 0; 0 1 0; 0 0 1]
  Transform Sensor : sm_lib/Frames and Transforms/Transform Sensor  MeasurementFrame=World  SenseAngle=on  SenseAxis=off  SenseAngle1=off  SenseAngle2=off  SenseAngle3=off  SenseQ=off  SenseR=off  SenseOmegaX=off  SenseOmegaY=on  SenseOmegaZ=off  SenseOmega1=off  SenseOmega2=off  SenseOmega3=off  SenseQDot=off  SenseRDot=off  SenseAlphaX=off  SenseAlphaY=off  SenseAlphaZ=off  SenseAlpha1=off  SenseAlpha2=off  SenseAlpha3=off  SenseQDDot=off  SenseRDDot=off  SenseX=off  SenseY=off  SenseZ=off  SenseRad=off  SenseAzim=off  SenseDist=off  SenseInc=off  SenseXDot=off  SenseYDot=off  SenseZDot=off  SenseRadDot=off  SenseAzimDot=off  SenseDistDot=off  SenseIncDot=off  SenseXDDot=off  SenseYDDot=off  SenseZDDot=off  SenseRadDDot=off  SenseAzimDDot=off  SenseDistDDot=off  SenseIncDDot=off
  World Frame : sm_lib/Frames and Transforms/World Frame
  Left Hip : PMIOPort  Side=Left
  Right Hip : PMIOPort  Port=2  Side=Left
  HATTop : PMIOPort  Port=3  Side=Right
  CG : PMIOPort  Port=4  Side=Right
  phiANDdphiHAT : Outport
  wires:
  Mux/1 -> phiANDdphiHAT/1
  PS-Simulink Converter1/1 -> Mux/2
  PS-Simulink Converter/1 -> Mux/1
  connections:
  HATTop/RConn1 -- HAT Center to Top/RConn1
  CG/RConn1 -- Inertia/RConn1 -- HAT CG/RConn1 -- HAT Center to CG/RConn1
  To: X-forward Y-Lateral Z-up/RConn1 -- Transform Sensor/RConn1
  Transform Sensor/RConn3 -- PS-Simulink Converter1/LConn1
  PS-Simulink Converter/LConn1 -- Transform Sensor/RConn2
  Transform Sensor/LConn1 -- World Frame/RConn1
  Right Hip/RConn1 -- Left Hip to Right Hip/RConn1
  HAT Center to Top/LConn1 -- Hip Solid/RConn1 -- HAT Center to CG/LConn1 -- Left Hip to Center/RConn1
  Left Hip to Right Hip/LConn1 -- Left Hip to Center/LConn1 -- Left Hip/RConn1 -- To: X-forward Y-Lateral Z-up/LConn1
